simulink model "debugECDD"  (Simulink 7.2)
settings: Solver=ode1  StartTime=0.0  StopTime=50  FixedStep=0.002  RelTol=1e-3
values from neighbouring files (symbols this model uses):
  a = param.a    [DSC_Control_Analysis.m]    (also in DSC_Control_Analysis_Exp.m; DSC_Speed_Control_Analysis.m; EmpiricalTireCurves.m = 1.35; FFW_Fx.m = sqrt(curvature/(2*clothoidLength)))
  b = 1.15    [EmpiricalTireCurves.m]
  Cfls = Cfl    [EC_params_nissan.m]
  Crls = Crl    [EC_params_nissan.m]
  Iz = param.Iz    [DSC_Control_Analysis.m]    (also in DSC_Control_Analysis_Exp.m; DSC_Speed_Control_Analysis.m; EmpiricalTireCurves.m = 1300)
  K = 10    [EC_params_nissan.m]
  Ks = -10    [EC_params_nissan.m]
  Ksl = -10    [EC_params_nissan.m]
  Kt = 40000    [EC_params_nissan.m]
  Ku = -40000    [EC_params_nissan.m]
  m = 1724    [EmpiricalTireCurves.m]
  mu_s = mu_p    (= 0.6)    [EC_params_nissan.m]    (also in EmpiricalTireCurves.m = 0.55)
  Ns = 10    [EC_params_nissan.m]
  q = 1    [EC_params_nissan.m]
undefined symbols (not defined in the file or in its folder): c, Cfl, Crl, dden, denafilt, dnum, filtera, filterb, h_roll, Ifalphaparam, numafilt, param, rfl, rfr, rrl, rrr, sglu, slimFxl, slimFxu, sliml, slimMll, slimMlr, slimMul, slimMur, slimu, steering_limit, tw_m, wc
libraries: simulink x15, xpclib x3, UserBlocks x1
(part 3 of 3)

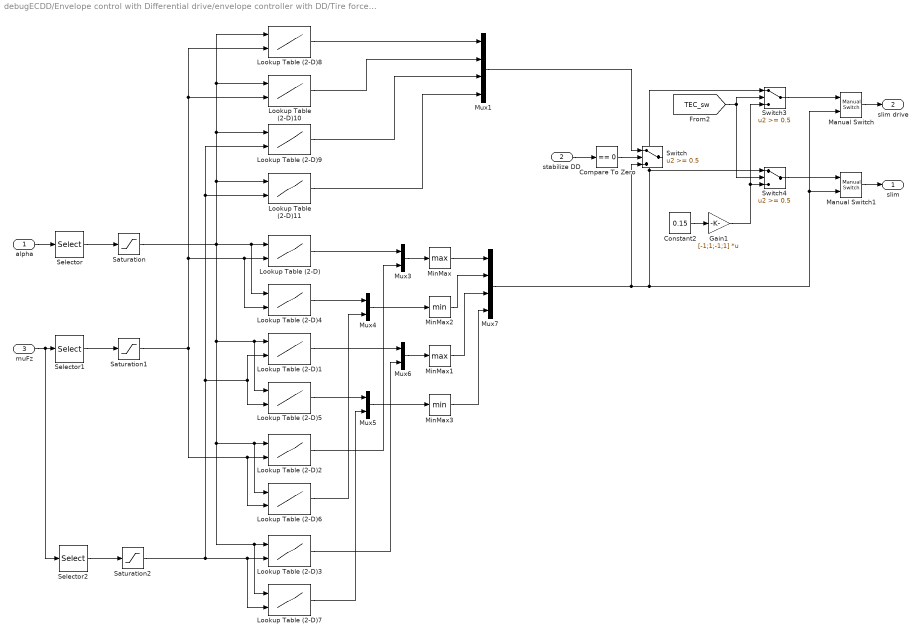
== system debugECDD/Envelope control with Differential drive/envelope controller with DD/Tire force control/limit_cal/slip_limit_cal1 ==
  alpha : Inport  OutDataType=sfix(16)  OutScaling=2^0
  stabilize DD : Inport  Port=2  OutDataType=sfix(16)  OutScaling=2^0
  muFz : Inport  Port=3  OutDataType=sfix(16)  OutScaling=2^0
  Compare To Zero : simulink/Logic and Bit Operations/Compare To Zero  SystemSampleTime=-1  relop===  LogicOutDataTypeMode=uint8  ZeroCross=off
  Constant2 : Constant  Value=0.15  OutDataType=sfix(16)  OutScaling=2^0
  Gain1 : Gain  Gain=[-1;1;-1;1]  Multiplication=Matrix(K*u)  ParameterDataType=sfix(16)  ParameterScaling=2^0  OutDataType=sfix(16)  OutScaling=2^0
  Lookup Table (2-D) : Lookup2D  RowIndex=limitcal_alphatbl  ColumnIndex=limitcal_muFztbl  Table=slimFxl  OutDataType=sfix(16)  OutScaling=2^0  SampleTime=0.002
  Lookup Table (2-D)1 : Lookup2D  RowIndex=limitcal_alphatbl  ColumnIndex=limitcal_muFztbl  Table=slimFxl  OutDataType=sfix(16)  OutScaling=2^0  SampleTime=0.002
  Lookup Table (2-D)10 : Lookup2D  RowIndex=limitcal_alphatbl  ColumnIndex=limitcal_muFztbl  Table=slimu  OutDataType=sfix(16)  OutScaling=2^0  SampleTime=0.002
  Lookup Table (2-D)11 : Lookup2D  RowIndex=limitcal_alphatbl  ColumnIndex=limitcal_muFztbl  Table=slimu  OutDataType=sfix(16)  OutScaling=2^0  SampleTime=0.002
  Lookup Table (2-D)2 : Lookup2D  RowIndex=limitcal_alphatbl  ColumnIndex=limitcal_muFztbl  Table=slimMll  OutDataType=sfix(16)  OutScaling=2^0  SampleTime=0.002
  Lookup Table (2-D)3 : Lookup2D  RowIndex=limitcal_alphatbl  ColumnIndex=limitcal_muFztbl  Table=slimMlr  OutDataType=sfix(16)  OutScaling=2^0  SampleTime=0.002
  Lookup Table (2-D)4 : Lookup2D  RowIndex=limitcal_alphatbl  ColumnIndex=limitcal_muFztbl  Table=slimFxu  OutDataType=sfix(16)  OutScaling=2^0  SampleTime=0.002
  Lookup Table (2-D)5 : Lookup2D  RowIndex=limitcal_alphatbl  ColumnIndex=limitcal_muFztbl  Table=slimFxu  OutDataType=sfix(16)  OutScaling=2^0  SampleTime=0.002
  Lookup Table (2-D)6 : Lookup2D  RowIndex=limitcal_alphatbl  ColumnIndex=limitcal_muFztbl  Table=slimMul  OutDataType=sfix(16)  OutScaling=2^0  SampleTime=0.002
  Lookup Table (2-D)7 : Lookup2D  RowIndex=limitcal_alphatbl  ColumnIndex=limitcal_muFztbl  Table=slimMur  OutDataType=sfix(16)  OutScaling=2^0  SampleTime=0.002
  Lookup Table (2-D)8 : Lookup2D  RowIndex=limitcal_alphatbl  ColumnIndex=limitcal_muFztbl  Table=sliml  OutDataType=sfix(16)  OutScaling=2^0  SampleTime=0.002
  Lookup Table (2-D)9 : Lookup2D  RowIndex=limitcal_alphatbl  ColumnIndex=limitcal_muFztbl  Table=sliml  OutDataType=sfix(16)  OutScaling=2^0  SampleTime=0.002
  Manual Switch : simulink/Signal Routing/Manual Switch  SystemSampleTime=-1  sw=1  action=0  varsize=off
  Manual Switch1 : simulink/Signal Routing/Manual Switch  SystemSampleTime=-1  sw=1  action=0  varsize=off
  MinMax : MinMax  Function=max  OutDataType=sfix(16)  OutScaling=2^0
  MinMax1 : MinMax  Function=max  OutDataType=sfix(16)  OutScaling=2^0
  MinMax2 : MinMax  OutDataType=sfix(16)  OutScaling=2^0
  MinMax3 : MinMax  OutDataType=sfix(16)  OutScaling=2^0
  Mux1 : Mux
  Mux{3..6} (4 alike) : Mux  Inputs=2
  Mux7 : Mux
  Saturation : Saturate  UpperLimit=40/180*pi  LowerLimit=-40/180*pi  OutDataType=sfix(16)  OutScaling=2^0
  Saturation1 : Saturate  UpperLimit=6000  LowerLimit=1  OutDataType=sfix(16)  OutScaling=2^0
  Saturation2 : Saturate  UpperLimit=6000  LowerLimit=1  OutDataType=sfix(16)  OutScaling=2^0
  Selector : Selector  InputPortWidth=2  IndexOptions=Index vector (dialog)  Indices=2  OutputSizes=1
  Selector1 : Selector  InputPortWidth=4  IndexOptions=Index vector (dialog)  Indices=3  OutputSizes=1
  Selector2 : Selector  InputPortWidth=4  IndexOptions=Index vector (dialog)  Indices=4  OutputSizes=1
  Switch : Switch  Threshold=0.5  OutDataType=sfix(16)  OutScaling=2^0
  Switch3 : Switch  Threshold=0.5
  Switch4 : Switch  Threshold=0.5
  slim : Outport  OutDataType=sfix(16)  OutScaling=2^0
  slim drive : Outport  Port=2  OutDataType=sfix(16)  OutScaling=2^0
  wires:
  Mux7/1 -> Switch/3, Manual Switch1/2, Manual Switch/2, Switch3/1, Switch4/1
  Lookup Table (2-D)11/1 -> Mux1/4
  Lookup Table (2-D)9/1 -> Mux1/3
  Lookup Table (2-D)10/1 -> Mux1/2
  Lookup Table (2-D)8/1 -> Mux1/1
  Compare To Zero/1 -> Switch/2
  alpha/1 -> Selector/1
  muFz/1 -> Selector1/1, Selector2/1
  Selector1/1 -> Saturation1/1
  Selector/1 -> Saturation/1
  Lookup Table (2-D)/1 -> Mux3/1
  Lookup Table (2-D)4/1 -> Mux4/1
  Lookup Table (2-D)1/1 -> Mux6/1
  Lookup Table (2-D)2/1 -> Mux3/2
  Lookup Table (2-D)6/1 -> Mux4/2
  Mux3/1 -> MinMax/1
  Mux6/1 -> MinMax1/1
  Mux4/1 -> MinMax2/1
  Mux5/1 -> MinMax3/1
  MinMax/1 -> Mux7/1
  MinMax2/1 -> Mux7/2
  MinMax1/1 -> Mux7/3
  MinMax3/1 -> Mux7/4
  Selector2/1 -> Saturation2/1
  Lookup Table (2-D)3/1 -> Mux6/2
  Lookup Table (2-D)7/1 -> Mux5/2
  Lookup Table (2-D)5/1 -> Mux5/1
  Saturation/1 -> Lookup Table (2-D)11/1, Lookup Table (2-D)9/1, Lookup Table (2-D)10/1, Lookup Table (2-D)8/1, Lookup Table (2-D)2/1, Lookup Table (2-D)6/1, Lookup Table (2-D)3/1, Lookup Table (2-D)7/1, Lookup Table (2-D)1/1, Lookup Table (2-D)5/1, Lookup Table (2-D)/1, Lookup Table (2-D)4/1
  Saturation1/1 -> Lookup Table (2-D)10/2, Lookup Table (2-D)8/2, Lookup Table (2-D)/2, Lookup Table (2-D)4/2, Lookup Table (2-D)2/2, Lookup Table (2-D)6/2
  Saturation2/1 -> Lookup Table (2-D)11/2, Lookup Table (2-D)9/2, Lookup Table (2-D)1/2, Lookup Table (2-D)5/2, Lookup Table (2-D)3/2, Lookup Table (2-D)7/2
  Constant2/1 -> Gain1/1
  stabilize DD/1 -> Compare To Zero/1
  [TEC_sw] -> Switch3/2, Switch4/2
  Gain1/1 -> Switch3/3, Switch4/3
  Manual Switch1/1 -> slim/1
  Manual Switch/1 -> slim drive/1
  Switch3/1 -> Manual Switch/1
  Switch4/1 -> Manual Switch1/1
  Mux1/1 -> Switch/1

== system debugECDD/Envelope control with Differential drive/envelope controller with DD/Tire force control/s_cal /prevent zero ==
  In1 : Inport  OutDataType=sfix(16)  OutScaling=2^0
  Abs : Abs
  Constant : Constant  Value=1/3.6  OutDataType=sfix(16)  OutScaling=2^0
  Product : Product  OutDataType=sfix(16)  OutScaling=2^0  RndMeth=Zero
  Relational Operator : RelationalOperator  Operator=>  LogicOutDataTypeMode=boolean  OutDataTypeStr=boolean
  Sign : Signum
  Switch : Switch  Threshold=0.5
  Switch1 : Switch  Threshold=0.5
  Unit Delay : UnitDelay  Orientation=left  X0=1  SampleTime=Ts
  Out1 : Outport  OutDataType=sfix(16)  OutScaling=2^0
  wires:
  Unit Delay/1 -> Switch1/3
  Switch1/1 -> Unit Delay/1, Product/2
  Product/1 -> Switch/3
  Sign/1 -> Switch1/1
  In1/1 -> Sign/1, Abs/1, Switch/1
  Abs/1 -> Relational Operator/1
  Constant/1 -> Product/1, Relational Operator/2
  Relational Operator/1 -> Switch1/2, Switch/2
  Switch/1 -> Out1/1

== system debugECDD/Envelope control with Differential drive/envelope controller with DD/Tire force control/s_cal /prevent zero1 ==
  In1 : Inport  OutDataType=sfix(16)  OutScaling=2^0
  Abs : Abs
  Constant : Constant  Value=1/3.6  OutDataType=sfix(16)  OutScaling=2^0
  Product : Product  OutDataType=sfix(16)  OutScaling=2^0  RndMeth=Zero
  Relational Operator : RelationalOperator  Operator=>  LogicOutDataTypeMode=boolean  OutDataTypeStr=boolean
  Sign : Signum
  Switch : Switch  Threshold=0.5
  Switch1 : Switch  Threshold=0.5
  Unit Delay : UnitDelay  Orientation=left  X0=1  SampleTime=Ts
  Out1 : Outport  OutDataType=sfix(16)  OutScaling=2^0
  wires:
  Switch/1 -> Out1/1
  Relational Operator/1 -> Switch/2, Switch1/2
  Constant/1 -> Relational Operator/2, Product/1
  Abs/1 -> Relational Operator/1
  In1/1 -> Switch/1, Abs/1, Sign/1
  Sign/1 -> Switch1/1
  Product/1 -> Switch/3
  Switch1/1 -> Product/2, Unit Delay/1
  Unit Delay/1 -> Switch1/3

== system debugECDD/Envelope control with Differential drive/envelope controller with DD/Tire force control/steering control/delta limit cal ==
  Vx : Inport  OutDataType=sfix(16)  OutScaling=2^0
  beta : Inport  Port=2  OutDataType=sfix(16)  OutScaling=2^0
  yaw rate : Inport  Port=3  OutDataType=sfix(16)  OutScaling=2^0
  aflim : Inport  Port=4  OutDataType=sfix(16)  OutScaling=2^0
  Fcn : Fcn  Expr=u[1]+a/u[3]*u[2]+u[4]  SampleTime=0.002
  Fcn1 : Fcn  Expr=u[1]+a/u[3]*u[2]-u[4]  SampleTime=0.002
  Mux : Mux
  upper lim : Outport  OutDataType=sfix(16)  OutScaling=2^0
  lower lim : Outport  Port=2  OutDataType=sfix(16)  OutScaling=2^0
  wires:
  Mux/1 -> Fcn1/1, Fcn/1
  Fcn/1 -> upper lim/1
  Fcn1/1 -> lower lim/1
  Vx/1 -> Mux/3
  aflim/1 -> Mux/4
  yaw rate/1 -> Mux/2
  beta/1 -> Mux/1

== system debugECDD/Envelope control with Differential drive/envelope controller with DD/vehicle motion control/EC/ay_limit_cal ==
  peak_force_hat : Inport  OutDataType=sfix(16)  OutScaling=2^0
  drive_trq : Inport  Port=2  OutDataType=sfix(16)  OutScaling=2^0
  ExpSW : Inport  Port=3  OutDataType=sfix(16)  OutScaling=2^0
  Constant : Constant  Value=0  OutDataType=sfix(16)  OutScaling=2^0
  Constant1 : Constant  Value=1.75  OutDataType=sfix(16)  OutScaling=2^0
  Demux : Demux
  Demux1 : Demux  Outputs=2
  Fcn : Fcn  Expr=u(1)*u(1)-u(2)*u(2)
  Fcn1 : Fcn  Expr=u(1)*u(1)-u(2)*u(2)
  Gain : Gain  Gain=1100  ParameterDataType=sfix(16)  ParameterScaling=2^0  OutDataType=sfix(16)  OutScaling=2^0
  Gain1 : Gain  Gain=400  ParameterDataType=sfix(16)  ParameterScaling=2^0  OutDataType=sfix(16)  OutScaling=2^0
  Gain2 : Gain  Gain=a  ParameterDataType=sfix(16)  ParameterScaling=2^0  OutDataType=sfix(16)  OutScaling=2^0
  Gain3 : Gain  Gain=b  ParameterDataType=sfix(16)  ParameterScaling=2^0  OutDataType=sfix(16)  OutScaling=2^0
  Gain4 : Gain  Gain=1+b/a  ParameterDataType=sfix(16)  ParameterScaling=2^0  OutDataType=sfix(16)  OutScaling=2^0
  Gain5 : Gain  Gain=1+a/b  ParameterDataType=sfix(16)  ParameterScaling=2^0  OutDataType=sfix(16)  OutScaling=2^0
  Gain6 : Gain  Gain=1/m  ParameterDataType=sfix(16)  ParameterScaling=2^0  OutDataType=sfix(16)  OutScaling=2^0
  Gain7 : Gain  Gain=1/rrl  ParameterDataType=sfix(16)  ParameterScaling=2^0  OutDataType=sfix(16)  OutScaling=2^0
  Gain8 : Gain  Gain=1/rrr  ParameterDataType=sfix(16)  ParameterScaling=2^0  OutDataType=sfix(16)  OutScaling=2^0
  Math Function : Math  Operator=sqrt  OutDataType=sfix(16)  OutScaling=2^0  SaturateOnIntegerOverflow=on
  Math Function1 : Math  Operator=sqrt  OutDataType=sfix(16)  OutScaling=2^0  SaturateOnIntegerOverflow=on
  MinMax : MinMax  Function=max  Inputs=2  OutDataType=sfix(16)  OutScaling=2^0
  MinMax1 : MinMax  Function=max  Inputs=2  OutDataType=sfix(16)  OutScaling=2^0
  Mux{,1,4..5} (4 alike) : Mux  Inputs=2
  Sum : Sum  Inputs=|++  OutDataType=sfix(16)  OutScaling=2^0
  Sum1 : Sum  Inputs=|+-  OutDataType=sfix(16)  OutScaling=2^0
  Sum2 : Sum  Inputs=|++  OutDataType=sfix(16)  OutScaling=2^0
  Sum3 : Sum  Inputs=-|+  OutDataType=sfix(16)  OutScaling=2^0
  Switch : Switch  OutDataType=sfix(16)  OutScaling=2^0
  Switch1 : Switch  OutDataType=sfix(16)  OutScaling=2^0
  Switch2 : Switch  Threshold=0.5  OutDataType=sfix(16)  OutScaling=2^0
  ay_limit : Outport  OutDataType=sfix(16)  OutScaling=2^0
  Force : Outport  Port=2  OutDataType=sfix(16)  OutScaling=2^0
  wires:
  peak_force_hat/1 -> Demux/1, Mux5/1
  Demux/1 -> Sum/1
  Demux/2 -> Sum/2
  Mux/1 -> Fcn/1
  Demux/3 -> Mux/1
  Demux/4 -> Mux1/1
  Demux1/1 -> Gain7/1
  Demux1/2 -> Gain8/1
  Mux1/1 -> Fcn1/1
  Fcn1/1 -> MinMax1/1
  Fcn/1 -> MinMax/1
  Constant/1 -> MinMax1/2, MinMax/2
  MinMax/1 -> Math Function/1
  MinMax1/1 -> Math Function1/1
  drive_trq/1 -> Sum1/1, Switch2/3
  Constant1/1 -> Sum1/2
  Sum1/1 -> Switch/2, Gain/1, Gain1/1
  Gain/1 -> Switch/1
  Gain1/1 -> Switch/3
  Math Function/1 -> Sum2/1
  Math Function1/1 -> Sum2/2
  Sum/1 -> Gain2/1, Gain5/1
  Sum2/1 -> Gain3/1, Gain4/1
  Sum3/1 -> Switch1/2
  Gain2/1 -> Sum3/1
  Gain3/1 -> Sum3/2
  Gain5/1 -> Switch1/1
  Gain4/1 -> Switch1/3
  Switch1/1 -> Gain6/1
  Gain6/1 -> ay_limit/1
  Switch2/1 -> Demux1/1
  Switch/1 -> Switch2/1
  ExpSW/1 -> Switch2/2
  Gain7/1 -> Mux/2, Mux4/1
  Gain8/1 -> Mux1/2, Mux4/2
  Mux4/1 -> Mux5/2
  Mux5/1 -> Force/1
